simulink model "moteur"  (R2022a)
settings: Solver=VariableStepAuto  StartTime=0.0  StopTime=10.0  RelTol=1e-3
settings Model: Creator=abbad12  LastModifiedBy=abbad12

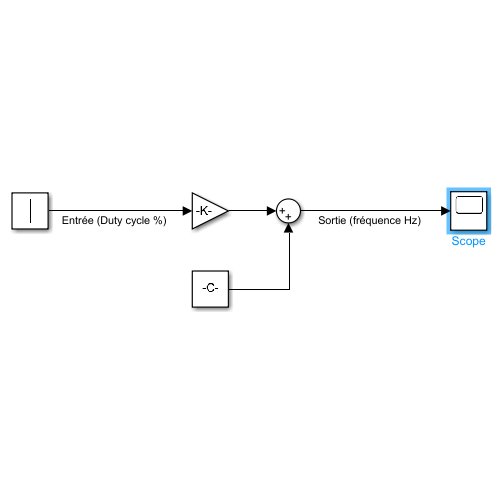
[thumbnail: Simulink's stored preview of the top-level diagram]
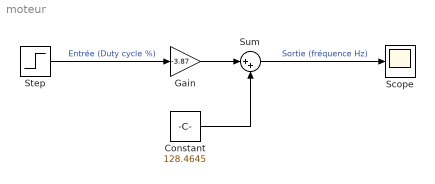
== system moteur ==
  Constant : Constant  Value=128.4645
  Gain : Gain  Gain=-3.87
  Scope : Scope
  Step : Step  Time=0.001  Before=11.79  After=2.72  SampleTime=0
  Sum : Sum  Inputs=|++
  wires:
  Sum/1 -> Scope/1  "Sortie (fréquence Hz)"
  Constant/1 -> Sum/2
  Gain/1 -> Sum/1
  Step/1 -> Gain/1  "Entrée (Duty cycle %)"
